simulink model "FPSO"  (R2024a)
settings: Solver=VariableStepAuto  StartTime=0  StopTime=(nit-1)*Ts  FixedStep=Ts  RelTol=1e-3
values from neighbouring files (symbols this model uses):
  L = Tuning_Parameters.scale.L    [Shell3x3.m]    (also in Shell7x5.m; WoodBerry.m; fpso.m; fpso_tuning.m)
  Ru = Tuning_Parameters.scale.Ru    [Shell3x3.m]    (also in Shell7x5.m; WoodBerry.m; fpso.m; fpso1.m = R(1:ny,1:ny))
  Rv = Tuning_Parameters.scale.Rv    [Shell3x3.m]    (also in Shell7x5.m; WoodBerry.m; fpso.m; fpso1.m = R(ny+1:end,ny+1:end))
  Ts = 4.0    (= 4)    [Shell3x3.m]    (also in Shell7x5.m; VanDeVusse_NMPC.m = 0.05; WoodBerry.m = 1; fpso.m = 20)
libraries: cstblocks x2, mpclib x1
settings Model: Creator=Sergio Castaño  LastModifiedBy=Sergio
settings SolverCC: AlgebraicLoopSolver=TrustRegion
settings DataIOCC: LimitDataPoints=on  ReturnWorkspaceOutputs=off
settings OptimizationCC: DefaultParameterBehavior=Inlined  UseFloatMulNetSlope=on  InlineInvariantSignals=on  EnhancedBackFolding=on  PassReuseOutputArgsAs=Individual arguments  EfficientFloat2IntCast=on  LifeSpan=inf  EfficientTunableParamExpr=on
settings DebuggingCC: ParameterTunabilityLossMsg=error  UnconnectedInputMsg=warning  UnconnectedOutputMsg=warning  UnconnectedLineMsg=warning  AllowSymbolicDim=off  SFUnexpectedBacktrackingDiag=warning  SFNoUnconditionalDefaultTransitionDiag=warning  SFExecutionAtInitializationDiag=none  ArithmeticOperatorsInVariantConditions=warning
settings HardwareCC: ProdBitPerSizeT=32  ProdBitPerPtrDiffT=32  ProdWordSize=32  ProdHWDeviceType=Specified
settings ModelReferenceCC: UpdateModelReferenceTargets=AssumeUpToDate  EnableRefExpFcnMdlSchedulingChecks=on  CheckModelReferenceTargetMessage=none  EnableParallelModelReferenceBuilds=on  PropagateSignalLabelsOutOfModel=off
settings SFSimCC: SimUseLocalCustomCode=off  MATLABDynamicMemAlloc=off  CustomCodeUndefinedFunction=UseInterfaceOnly
settings RTWCC: Description=Embedded Coder  SystemTargetFile=ert.tlc  TemplateMakefile=ert_default_tmf  GenerateReport=on  RTWUseLocalCustomCode=off  IncludeHyperlinkInReport=on  LaunchReport=on  GenerateTraceInfo=on  GenerateTraceReport=on  GenerateTraceReportSl=on  GenerateTraceReportSf=on  GenerateTraceReportEml=on  GPUComputeCapability=3.5  DLArmComputeVersion=19.05
settings CodeAppCC: ForceParamTrailComments=on  IgnoreCustomStorageClasses=off  OperatorAnnotations=on  SimulinkDataObjDesc=on  SFDataObjDesc=on  InsertBlockDesc=on  StateflowObjectComments=on
settings ERTTargetCC: GenerateSampleERTMain=on  SupportContinuousTime=on  InlinedParameterPlacement=NonHierarchical  ERTCustomFileTemplate=example_file_process.tlc
settings ConfigComp: CovMetricSettings=dw  CovSaveCumulativeToWorkspaceVar=on  CovSaveSingleToWorkspaceVar=on  CovExternalEMLEnable=off

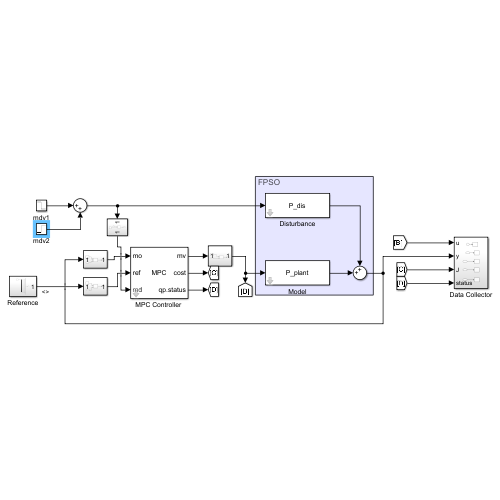
[thumbnail: Simulink's stored preview of the top-level diagram]
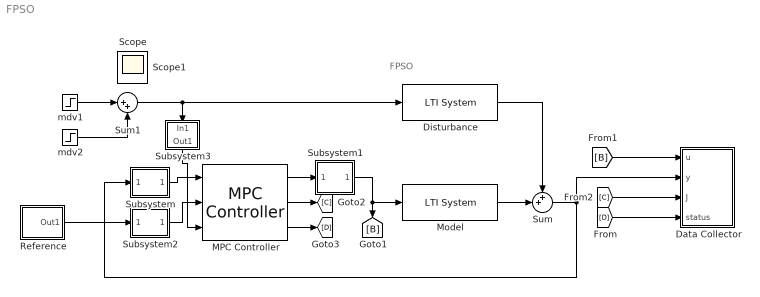
== system FPSO ==
  note: FPSO
  Data Collector : Subsystem
  Disturbance : cstblocks/LTI System  sys=P_dis  IC=[]  PadeOrder=0
  "MPC Controller " : mpclib/MPC Controller  SCDEnableBlockLinearizationSpecification=on  mpcobj=mpc_toolbox  is_multiple=0  enable_value=0  return_u0=off  updateMPCinCallerWorkspace=on  md_inport=on  mv_inport=off  uref_inport=off  return_cost=on  return_mvseq=off  return_qpstatus=on  return_xseq=off  return_state=off  return_ovseq=off  state_inport=off  umin_inport=off  umax_inport=off  ymin_inport=off  ymax_inport=off  cc_inport=off  ywt_inport=off  uwt_inport=off  duwt_inport=off  rhoeps_inport=off  pm_inport=off  MaximumP=10  HorizonChoice=FixedHorizon  n_ts=20  n_p=9  n_mv=3  n_md=1  n_ud=0  n_mo=14  n_uo=0  BlockDataType=double  SampleTimeInherited=off  switch_inport=off
  Model : cstblocks/LTI System  sys=P_plant  IC=[]  PadeOrder=0
  Reference : Subsystem
  Subsystem : Subsystem
  Subsystem1 : Subsystem
  Subsystem2 : Subsystem
  Subsystem3 : Subsystem
  Sum : Sum  Inputs=++|
  Sum1 : Sum  Inputs=|++
  mdv1 : Step  Time=500  After=-5  SampleTime=0
  mdv2 : Step  Time=2000  After=10  SampleTime=0
  Scope : Scope
  Scope1 : Scope
  wires:
  "MPC Controller "/1 -> Subsystem1/1(In1)
  Model/1 -> Sum/2
  Sum/1 -> Data Collector/2(y), Subsystem/1(In1)
  Subsystem/1(Out1) -> "MPC Controller "/1
  Subsystem2/1(Out1) -> "MPC Controller "/2
  Subsystem1/1(Out1) -> [B], Model/1
  Reference/1(Out1) -> Subsystem2/1(In1)
  [B] -> Data Collector/1(u)
  Subsystem3/1(Out1) -> "MPC Controller "/3
  Disturbance/1 -> Sum/1
  mdv1/1 -> Sum1/1
  mdv2/1 -> Sum1/2
  Sum1/1 -> Subsystem3/1(In1), Disturbance/1
  "MPC Controller "/2 -> [C]
  "MPC Controller "/3 -> [D]
  [D] -> Data Collector/4(status)
  [C] -> Data Collector/3(J)

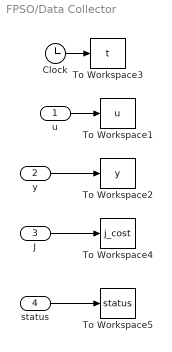
== system FPSO/Data Collector ==
  u : Inport
  y : Inport  Port=2
  J : Inport  Port=3
  status : Inport  Port=4
  Clock : Clock
  To Workspace1 : ToWorkspace  VariableName=u  SampleTime=Ts
  To Workspace2 : ToWorkspace  VariableName=y  SampleTime=Ts
  To Workspace3 : ToWorkspace  VariableName=t  SampleTime=Ts
  To Workspace4 : ToWorkspace  VariableName=j_cost  SampleTime=Ts
  To Workspace5 : ToWorkspace  VariableName=status  SampleTime=Ts
  wires:
  y/1 -> To Workspace2/1
  u/1 -> To Workspace1/1
  Clock/1 -> To Workspace3/1
  J/1 -> To Workspace4/1
  status/1 -> To Workspace5/1

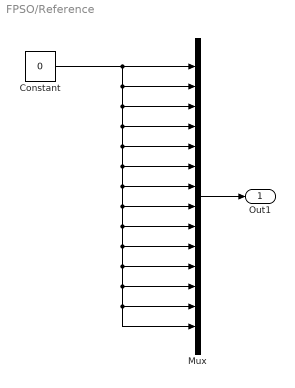
== system FPSO/Reference ==
  Constant : Constant  Value=0
  Mux : Mux  Inputs=14
  Out1 : Outport  VectorParamsAs1DForOutWhenUnconnected=off
  wires:
  Mux/1 -> Out1/1
  Constant/1 -> Mux/2, Mux/3, Mux/4, Mux/5, Mux/6, Mux/7, Mux/8, Mux/9, Mux/10, Mux/11, Mux/12, Mux/13, Mux/14, Mux/1

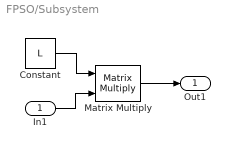
== system FPSO/Subsystem ==
  In1 : Inport
  Constant : Constant  Value=L
  Matrix Multiply : Product  Multiplication=Matrix(*)
  Out1 : Outport
  wires:
  Matrix Multiply/1 -> Out1/1
  In1/1 -> Matrix Multiply/2
  Constant/1 -> Matrix Multiply/1

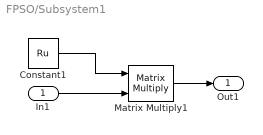
== system FPSO/Subsystem1 ==
  In1 : Inport
  Constant1 : Constant  Value=Ru
  Matrix Multiply1 : Product  Multiplication=Matrix(*)
  Out1 : Outport
  wires:
  Matrix Multiply1/1 -> Out1/1
  In1/1 -> Matrix Multiply1/2
  Constant1/1 -> Matrix Multiply1/1

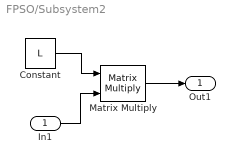
== system FPSO/Subsystem2 ==
  In1 : Inport
  Constant : Constant  Value=L
  Matrix Multiply : Product  Multiplication=Matrix(*)
  Out1 : Outport
  wires:
  Matrix Multiply/1 -> Out1/1
  Constant/1 -> Matrix Multiply/1
  In1/1 -> Matrix Multiply/2

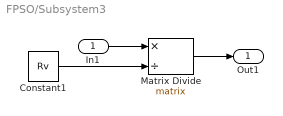
== system FPSO/Subsystem3 ==
  In1 : Inport
  Constant1 : Constant  Value=Rv
  Matrix Divide : Product  Inputs=*/  Multiplication=Matrix(*)
  Out1 : Outport
  wires:
  Constant1/1 -> Matrix Divide/2
  In1/1 -> Matrix Divide/1
  Matrix Divide/1 -> Out1/1
